simulink library "INT_CEngDsT_DD"  (R2016b)
settings: Solver=VariableStepAuto  StartTime=0.0  StopTime=10.0  RelTol=1e-3
settings Model: Creator=Administrator  LastModifiedBy=Administrator

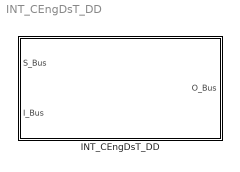
== system INT_CEngDsT_DD ==
  INT_CEngDsT_DD : Subsystem

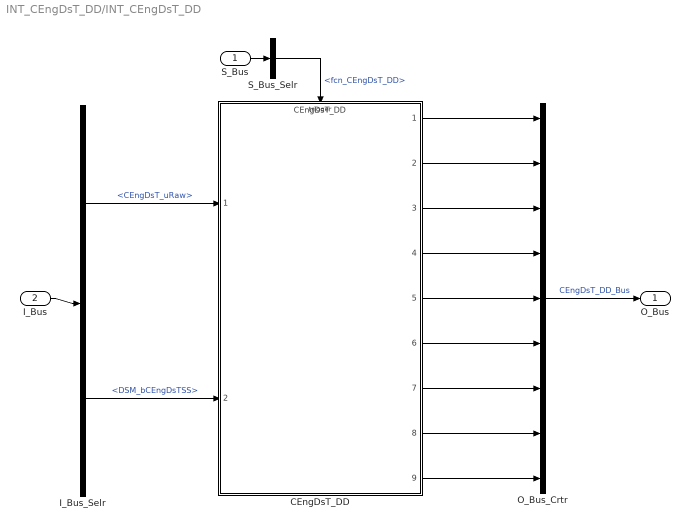
== system INT_CEngDsT_DD/INT_CEngDsT_DD ==
  S_Bus : Inport
  I_Bus : Inport  Port=2
  CEngDsT_DD : ModelReference  ModelNameDialog=CEngDsT_DD  SimulationMode=Normal  ModelReferenceVersion=1.15  TriggerPortName=function  TriggerPortTriggerType=function-call  TriggerPortStatesWhenEnabling=held
  I_Bus_Selr : BusSelector  OutputSignals=CEngDsT_uRaw,DSM_bCEngDsTSS
  O_Bus_Crtr : BusCreator  Inputs=9
  S_Bus_Selr : BusSelector  OutputSignals=fcn_CEngDsT_DD
  O_Bus : Outport
  wires:
  S_Bus_Selr/1 -> CEngDsT_DD/Trigger  "<fcn_CEngDsT_DD>"
  S_Bus/1 -> S_Bus_Selr/1
  I_Bus/1 -> I_Bus_Selr/1
  I_Bus_Selr/1 -> CEngDsT_DD/1  "<CEngDsT_uRaw>"
  I_Bus_Selr/2 -> CEngDsT_DD/2  "<DSM_bCEngDsTSS>"
  O_Bus_Crtr/1 -> O_Bus/1  "CEngDsT_DD_Bus"
  CEngDsT_DD/1 -> O_Bus_Crtr/1
  CEngDsT_DD/2 -> O_Bus_Crtr/2
  CEngDsT_DD/3 -> O_Bus_Crtr/3
  CEngDsT_DD/4 -> O_Bus_Crtr/4
  CEngDsT_DD/5 -> O_Bus_Crtr/5
  CEngDsT_DD/6 -> O_Bus_Crtr/6
  CEngDsT_DD/7 -> O_Bus_Crtr/7
  CEngDsT_DD/8 -> O_Bus_Crtr/8
  CEngDsT_DD/9 -> O_Bus_Crtr/9
